simulink model "fz8_3"  (R2014a)
settings: Solver=ode45  StartTime=0.0  StopTime=10.0  RelTol=1e-3
values from neighbouring files (symbols this model uses):
  SymbolRate = 50000    [eg8_3.m]
undefined symbols (not defined in the file or in its folder): gfprimfd
libraries: commdigbbndpm3 x4, commchan3 x2, commsink2 x2, commblkcod2 x2, dspsigops x1, commrandsrc2 x1
settings Model: Creator=tzb  LastModifiedBy=tzb
settings DebuggingCC: SolverPrmCheckMsg=none

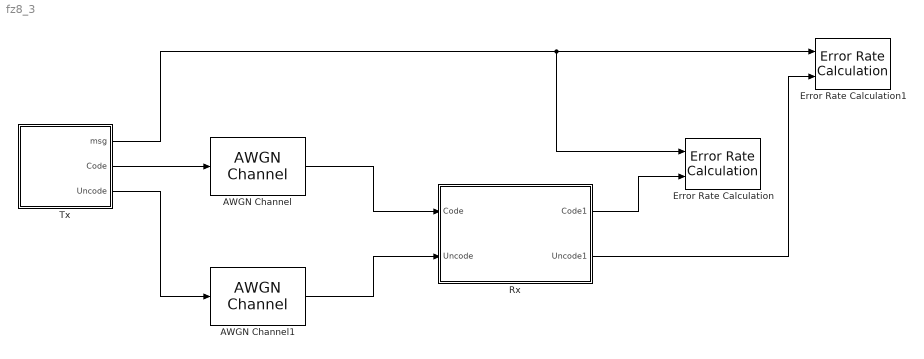
== system fz8_3 ==
  AWGN Channel : commchan3/AWGN Channel  InputProcessing=Columns as channels (frame based)  seed=67  noiseMode="Signal to noise ratio  (Eb/No)"  EbNodB=SNR  EsNodB=10  SNRdB=10  bitsPerSym=2  Ps=1  Tsym=1/SymbolRate  variance=1
  AWGN Channel1 : commchan3/AWGN Channel  InputProcessing=Columns as channels (frame based)  seed=67  noiseMode="Signal to noise ratio  (Eb/No)"  EbNodB=SNR  EsNodB=10  SNRdB=10  bitsPerSym=2  Ps=1  Tsym=1/SymbolRate  variance=1
  Error Rate Calculation : commsink2/Error Rate Calculation  N=8  st_delay=0  cp_mode=Entire frame  subframe=[]  PMode=Workspace  WsName=BER2  RsMode2=off  stop=off  numErr=100  maxBits=1e6
  Error Rate Calculation1 : commsink2/Error Rate Calculation  N=0  st_delay=0  cp_mode=Entire frame  subframe=[]  PMode=Workspace  WsName=BER1  RsMode2=off  stop=off  numErr=100  maxBits=1e6
  Rx : Subsystem
  Tx : Subsystem
  wires:
  Tx/2(Code) -> AWGN Channel/1
  AWGN Channel/1 -> Rx/1(Code)
  Tx/3(Uncode) -> AWGN Channel1/1
  AWGN Channel1/1 -> Rx/2(Uncode)
  Tx/1(msg) -> Error Rate Calculation/1, Error Rate Calculation1/1
  Rx/1(Code1) -> Error Rate Calculation/2
  Rx/2(Uncode1) -> Error Rate Calculation1/2

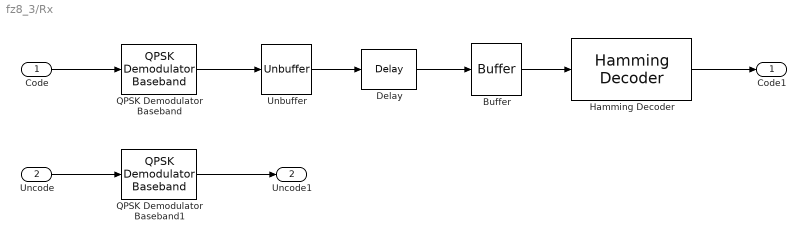
== system fz8_3/Rx ==
  Code : Inport
  Uncode : Inport  Port=2
  Buffer : Buffer  N=7  TreatMby1Signals=One channel
  Delay : dspsigops/Delay  InputProcessing=Columns as channels (frame based)  dly_unit=Samples  delay=5  ic_detail=off  dif_ic_for_ch=off  dif_ic_for_dly=off  ic=0  reset_popup=None
  Hamming Decoder : commblkcod2/Hamming Decoder  n=7  k=gfprimfd(3,'min')
  QPSK Demodulator Baseband : commdigbbndpm3/QPSK Demodulator Baseband  Ph=pi/4  Dec=Gray  OutType=Bit  DecType=Hard decision  VarSource=Dialog  Variance=1  outDtype1=Inherit via internal rule  outDtype2=Inherit via internal rule  derotateFactorWordLen=16
  QPSK Demodulator Baseband1 : commdigbbndpm3/QPSK Demodulator Baseband  Ph=pi/4  Dec=Gray  OutType=Bit  DecType=Hard decision  VarSource=Dialog  Variance=1  outDtype1=Inherit via internal rule  outDtype2=Inherit via internal rule  derotateFactorWordLen=16
  Unbuffer : Unbuffer  SampleBasedProcessing=Same as frame based
  Code1 : Outport
  Uncode1 : Outport  Port=2
  wires:
  Unbuffer/1 -> Delay/1
  Buffer/1 -> Hamming Decoder/1
  QPSK Demodulator Baseband/1 -> Unbuffer/1
  Code/1 -> QPSK Demodulator Baseband/1
  Delay/1 -> Buffer/1
  Hamming Decoder/1 -> Code1/1
  Uncode/1 -> QPSK Demodulator Baseband1/1
  QPSK Demodulator Baseband1/1 -> Uncode1/1

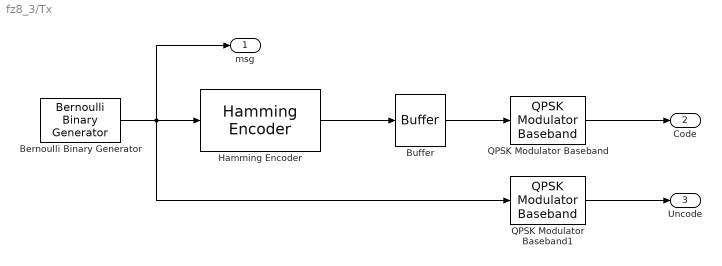
== system fz8_3/Tx ==
  Bernoulli Binary Generator : commrandsrc2/Bernoulli Binary Generator  P=0.5  seed=61  Ts=1/(2*SymbolRate)  frameBased=on  sampPerFrame=4  orient=off  outDataType=double
  Buffer : Buffer  N=2  TreatMby1Signals=One channel
  Hamming Encoder : commblkcod2/Hamming Encoder  n=7  k=gfprimfd(3,'min')
  QPSK Modulator Baseband : commdigbbndpm3/QPSK Modulator Baseband  InType=Bit  Enc=Gray  Ph=pi/4  outDtype=double  outWordLen=16  outUDDataType=sfix(16)  outFracLenMode=Best precision  outFracLen=15
  QPSK Modulator Baseband1 : commdigbbndpm3/QPSK Modulator Baseband  InType=Bit  Enc=Gray  Ph=pi/4  outDtype=double  outWordLen=16  outUDDataType=sfix(16)  outFracLenMode=Best precision  outFracLen=15
  msg : Outport
  Code : Outport  Port=2
  Uncode : Outport  Port=3
  wires:
  Hamming Encoder/1 -> Buffer/1
  QPSK Modulator Baseband1/1 -> Uncode/1
  Bernoulli Binary Generator/1 -> msg/1, QPSK Modulator Baseband1/1, Hamming Encoder/1
  QPSK Modulator Baseband/1 -> Code/1
  Buffer/1 -> QPSK Modulator Baseband/1
